simulink model "exp2"  (R2022a)
settings: Solver=VariableStepAuto  StartTime=0.0  StopTime=10.0  RelTol=1e-3
settings Model: Creator=Guilherme  LastModifiedBy=Guilherme

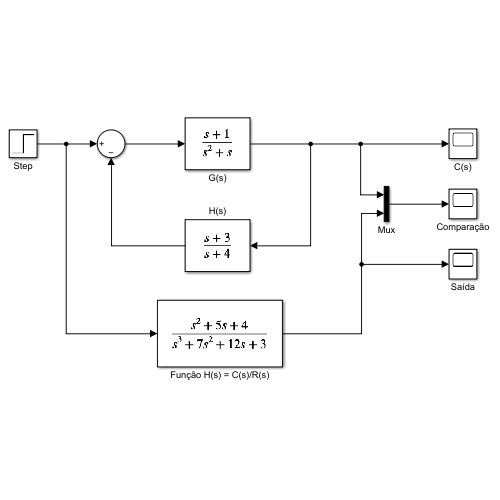
[thumbnail: Simulink's stored preview of the top-level diagram]
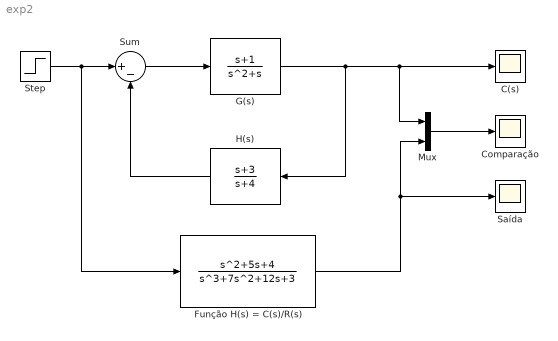
== system exp2 ==
  C(s) : Scope
  Comparação : Scope
  Função H(s) = C(s)/R(s) : TransferFcn  Numerator=[1 5 4]  Denominator=[1 7 12 3]
  G(s) : TransferFcn  Numerator=[1 1]  Denominator=[1 1 0 ]
  H(s) : TransferFcn  Numerator=[1 3]  Denominator=[1 4]
  Mux : Mux  Inputs=2
  Saída : Scope
  Step : Step  SampleTime=0
  Sum : Sum  Inputs=|+-
  wires:
  G(s)/1 -> C(s)/1, Mux/1, H(s)/1
  H(s)/1 -> Sum/2
  Sum/1 -> G(s)/1
  Step/1 -> Função H(s) = C(s)/R(s)/1, Sum/1
  Função H(s) = C(s)/R(s)/1 -> Mux/2, Saída/1
  Mux/1 -> Comparação/1
